simulink model "in_gps_estimation"  (R2021b)
settings: Solver=ode4  StartTime=0.0  StopTime=30  FixedStep=ts  RelTol=1e-3
values from neighbouring files (symbols this model uses):
  ts = 0.0005    [dc_motor_ingps.m]    (also in dc_sim_inpgps.m; in_gps_est.m; untitled.m)
undefined symbols (not defined in the file or in its folder): BlockInfo, ParamInfo, PortInfo, TimeInfo
libraries: simulink x4
settings Model: SimulationMode=rapid-accelerator  Creator=JongBeom  LastModifiedBy=JongBeom
settings DataIOCC: ReturnWorkspaceOutputs=off

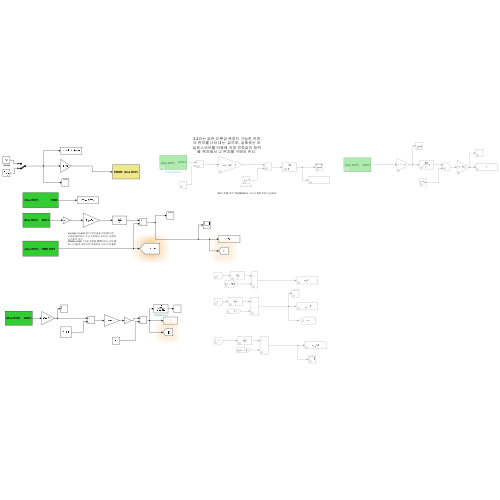
[thumbnail: Simulink's stored preview of the top-level diagram]
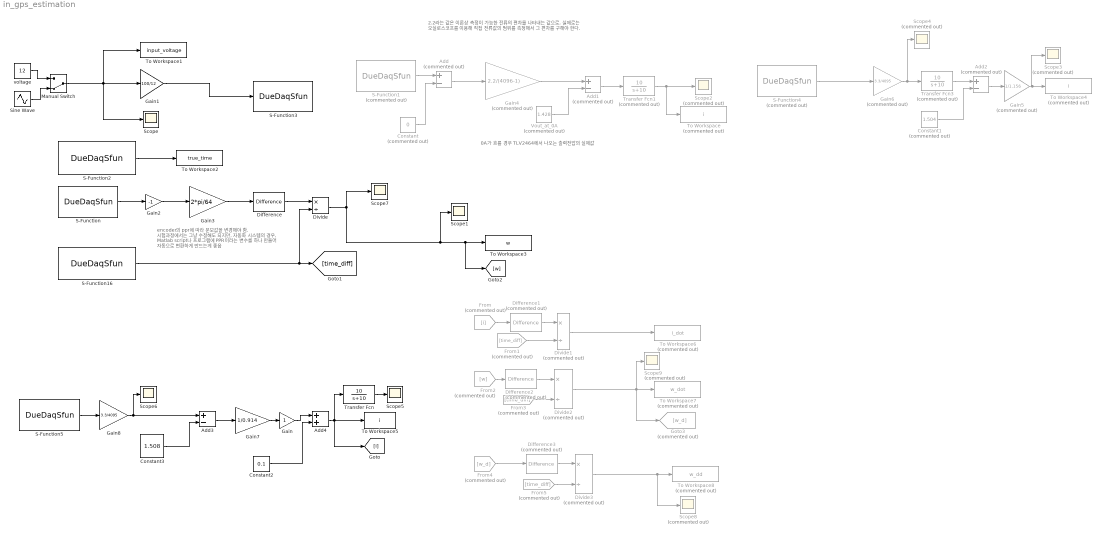
== system in_gps_estimation ==
  note: 0A가 흐를 경우 TLV2464에서 나오는 출력전압의 실제값
  note: 2.2라는 값은 이론상 측정이 가능한 전류의 편차를 나타내는 값으로, 실제로는 오실로스코프를 이용해 직접 전류값의 범위를 측정해서 그 편차를 구해야 한다.
  note: encoder의 ppr에 따라 분모값을 변경해야 함.
      | 시험과정에서는 그냥 수정해도 되지만, 자동화 시스템의 경우,
      | Matlab script나 프로그램에 PPR이라는 변수를 하나 만들어 자동으로 변환하게 만드는게 좋음
  Add : Sum  Commented=on  Inputs=+-
  Add1 : Sum  Commented=on  Inputs=+-
  Add2 : Sum  Commented=on  Inputs=+-
  Add3 : Sum  Inputs=+-
  Add4 : Sum
  Constant : Constant  Commented=on  Value=0
  Constant1 : Constant  Commented=on  Value=1.504
  Constant2 : Constant  Value=0.1
  Constant3 : Constant  Value=1.508
  Difference : simulink/Discrete/Difference  ICPrevInput=0.0  OutMin=[]  OutMax=[]  OutDataType=fixdt(1, 16)  OutScaling=2^-10  DoSatur=off
  Difference1 : simulink/Discrete/Difference  Commented=on  ICPrevInput=0.0  OutMin=[]  OutMax=[]  OutDataType=fixdt(1, 16)  OutScaling=2^-10  DoSatur=off
  Difference2 : simulink/Discrete/Difference  Commented=on  ICPrevInput=0.0  OutMin=[]  OutMax=[]  OutDataType=fixdt(1, 16)  OutScaling=2^-10  DoSatur=off
  Difference3 : simulink/Discrete/Difference  Commented=on  ICPrevInput=0.0  OutMin=[]  OutMax=[]  OutDataType=fixdt(1, 16)  OutScaling=2^-10  DoSatur=off
  Divide : Product  Inputs=*/
  Divide1 : Product  Commented=on  Inputs=*/
  Divide2 : Product  Commented=on  Inputs=*/
  Divide3 : Product  Commented=on  Inputs=*/
  From : From  Commented=on  GotoTag=i
  From1 : From  Commented=on  GotoTag=time_diff
  From2 : From  Commented=on  GotoTag=w
  From3 : From  Commented=on  GotoTag=time_diff
  From4 : From  Commented=on  GotoTag=w_d
  From5 : From  Commented=on  GotoTag=time_diff
  Gain : Gain
  Gain1 : Gain  Gain=100/12
  Gain2 : Gain  Gain=-1
  Gain3 : Gain  Gain=2*pi/64
  Gain4 : Gain  Commented=on  Gain=2.2/(4096-1)
  Gain5 : Gain  Commented=on  Gain=1/1.156
  Gain6 : Gain  Commented=on  Gain=3.3/4095
  Gain7 : Gain  Gain=1/0.914
  Gain8 : Gain  Gain=3.3/4095
  Goto3 : Goto  Commented=on  GotoTag=w_d
  Manual Switch : ManualSwitch  CurrentSetting=0
  S-Function : S-Function  FunctionName=DueDaqSfun  Parameters=TimeInfo,BlockInfo,ParamInfo,PortInfo  SFunctionDeploymentMode=off  EnableBusSupport=off  mask(Encoder Block){channel=1}
      mask prompts: channel "Channel Number"
      mask help: Receive encoder count value from Arduino Due
      mask init:
      | DueDaqRcp_Encoder_callback;
      mask TypeOptions channel: 0 | 1
      mask Display:
      | color('black');text(0.05,0.5,'(Due RCP)','horizontalalignment','left');
      | color('black');port_label('output', 1,  ' ENC1');
  S-Function1 : S-Function  Commented=on  FunctionName=DueDaqSfun  Parameters=TimeInfo,BlockInfo,ParamInfo,PortInfo  SFunctionDeploymentMode=off  EnableBusSupport=off  mask(ADC Block){channel=1}
      mask prompts: channel "Channel Number"
      mask help: Receive ADC data from Arduino Due
      mask init:
      | DueDaqRcp_ADC_callback;
      mask TypeOptions channel: 0 | 1 | 2 | 3 | 4 | 5 | 6 | 7
      mask Display:
      | color('black');text(0.05,0.5,'(Due RCP)','horizontalalignment','left');
      | color('black');port_label('output', 1,  ' ADC1')
  S-Function16 : S-Function  FunctionName=DueDaqSfun  Parameters=TimeInfo,BlockInfo,ParamInfo,PortInfo  SFunctionDeploymentMode=off  EnableBusSupport=off  mask(Time Data Block){time_data_type=Time Difference}
      mask prompts: time_data_type "Time Data Type"
      mask help: Receive time-related data from Arduino Due
      mask init:
      | DueDaqRcp_TimeDiff_callback;
      mask TypeOptions time_data_type: Time | Time Difference
      mask Display:
      | color('black');text(0.05,0.5,'(Due RCP)','horizontalalignment','left');
      | color('black');port_label('output', 1,  ' TIME DIFF   ')
  S-Function2 : S-Function  FunctionName=DueDaqSfun  Parameters=TimeInfo,BlockInfo,ParamInfo,PortInfo  SFunctionDeploymentMode=off  EnableBusSupport=off  mask(Time Data Block){time_data_type=Time}
      mask prompts: time_data_type "Time Data Type"
      mask help: Receive time-related data from Arduino Due
      mask init:
      | DueDaqRcp_TimeDiff_callback;
      mask TypeOptions time_data_type: Time | Time Difference
      mask Display:
      | color('black');text(0.05,0.5,'(Due RCP)','horizontalalignment','left');
      | color('black');port_label('output', 1,  ' TIME')
  S-Function3 : S-Function  FunctionName=DueDaqSfun  Parameters=TimeInfo,BlockInfo,ParamInfo,PortInfo  SFunctionDeploymentMode=off  EnableBusSupport=off  mask(PWM Block){channel=0, method=PWM/Direction, sync=off, freq=20, dead_time=3}
      mask prompts: channel "Channel Number"; sync "Synchronization with Channel 0"; freq "Frequency (KHz)"; dead_time "Dead Time"
      mask help: Send PWM information to Arduino Due
      mask init:
      | DueDaqRcp_PWM_callback;
      mask TypeOptions channel: 0 | 1 | 2 | 3 | 4 | 5
      mask Callback channel: DueDaqRcp_PWM_callback;
      mask TypeOptions method: PWM/Direction | Complementary PWM
      mask Callback method: DueDaqRcp_PWM_callback;
      mask TypeOptions freq: 1 | 10 | 20
      mask Display:
      | color('black');text(0.95,0.5,'(Due RCP)','horizontalalignment','right');
      | color('black');port_label('input', 1,  ' PWM0')
  S-Function4 : S-Function  Commented=on  FunctionName=DueDaqSfun  Parameters=TimeInfo,BlockInfo,ParamInfo,PortInfo  SFunctionDeploymentMode=off  EnableBusSupport=off  mask(ADC Block){channel=1}
      mask prompts: channel "Channel Number"
      mask help: Receive ADC data from Arduino Due
      mask init:
      | DueDaqRcp_ADC_callback;
      mask TypeOptions channel: 0 | 1 | 2 | 3 | 4 | 5 | 6 | 7
      mask Display:
      | color('black');text(0.05,0.5,'(Due RCP)','horizontalalignment','left');
      | color('black');port_label('output', 1,  ' ADC1')
  S-Function5 : S-Function  FunctionName=DueDaqSfun  Parameters=TimeInfo,BlockInfo,ParamInfo,PortInfo  SFunctionDeploymentMode=off  EnableBusSupport=off  mask(ADC Block){channel=1}
      mask prompts: channel "Channel Number"
      mask help: Receive ADC data from Arduino Due
      mask init:
      | DueDaqRcp_ADC_callback;
      mask TypeOptions channel: 0 | 1 | 2 | 3 | 4 | 5 | 6 | 7
      mask Display:
      | color('black');text(0.05,0.5,'(Due RCP)','horizontalalignment','left');
      | color('black');port_label('output', 1,  ' ADC1')
  Scope{,1,5..7} (5 alike) : Scope
  Scope{2..4,8..9} (5 alike) : Scope  Commented=on
  Sine Wave : Sin  Amplitude=9  SampleTime=0
  To Workspace : ToWorkspace  Commented=on  VariableName=i  SampleTime=-1
  To Workspace1 : ToWorkspace  VariableName=input_voltage  SampleTime=-1
  To Workspace2 : ToWorkspace  VariableName=true_time  SampleTime=-1
  To Workspace3 : ToWorkspace  VariableName=w  SampleTime=-1
  To Workspace4 : ToWorkspace  Commented=on  VariableName=i  SampleTime=-1
  To Workspace5 : ToWorkspace  VariableName=i  SampleTime=-1
  To Workspace6 : ToWorkspace  Commented=on  VariableName=i_dot  SampleTime=-1
  To Workspace7 : ToWorkspace  Commented=on  VariableName=w_dot  SampleTime=-1
  To Workspace8 : ToWorkspace  Commented=on  VariableName=w_dd  SampleTime=-1
  Transfer Fcn : TransferFcn  Numerator=[10]  Denominator=[1 10]
  Transfer Fcn1 : TransferFcn  Commented=on  Numerator=[10]  Denominator=[1 10]
  Transfer Fcn3 : TransferFcn  Commented=on  Numerator=[10]  Denominator=[1 10]
  Vout_at_0A : Constant  Commented=on  Value=1.428
  voltage : Constant  Value=12  SampleTime=ts
  wires:
  Gain2/1 -> Gain3/1
  S-Function/1 -> Gain2/1
  Gain3/1 -> Difference/1
  Difference/1 -> Divide/1
  S-Function16/1 -> Divide/2, [time_diff]
  S-Function1/1 -> Add/1
  Add/1 -> Gain4/1
  Constant/1 -> Add/2
  Gain4/1 -> Add1/1
  Vout_at_0A/1 -> Add1/2
  Add1/1 -> Transfer Fcn1/1
  Transfer Fcn1/1 -> To Workspace/1, Scope2/1
  S-Function2/1 -> To Workspace2/1
  Divide/1 -> Scope1/1, [w], To Workspace3/1, Scope7/1
  Constant1/1 -> Add2/2
  Transfer Fcn3/1 -> Add2/1
  Gain5/1 -> To Workspace4/1, Scope3/1
  Gain6/1 -> Scope4/1, Transfer Fcn3/1
  Add2/1 -> Gain5/1
  S-Function4/1 -> Gain6/1
  Add3/1 -> Gain7/1
  Gain8/1 -> Add3/1, Scope6/1
  S-Function5/1 -> Gain8/1
  Constant3/1 -> Add3/2
  Gain7/1 -> Gain/1
  From/1 -> Difference1/1
  From1/1 -> Divide1/2
  From2/1 -> Difference2/1
  From3/1 -> Divide2/2
  Difference1/1 -> Divide1/1
  Difference2/1 -> Divide2/1
  Gain1/1 -> S-Function3/1
  Divide1/1 -> To Workspace6/1
  Divide2/1 -> Scope9/1, Goto3/1, To Workspace7/1
  Transfer Fcn/1 -> Scope5/1
  Divide3/1 -> Scope8/1, To Workspace8/1
  Difference3/1 -> Divide3/1
  From5/1 -> Divide3/2
  From4/1 -> Difference3/1
  voltage/1 -> Manual Switch/1
  Manual Switch/1 -> Scope/1, Gain1/1, To Workspace1/1
  Constant2/1 -> Add4/2
  Gain/1 -> Add4/1
  Add4/1 -> [i], Transfer Fcn/1, To Workspace5/1
  Sine Wave/1 -> Manual Switch/2
